simulink model "dynamicsquat"  (R2023a)
settings: Solver=VariableStepAuto  StartTime=0.0  StopTime=stoptimetotal  RelTol=1e-3
values from neighbouring files (symbols this model uses):
  battery = load('params/battery_Tattu.mat').battery    [runDetailedT18Model.m]
  IC = load('params/initialcond/IC_HoverAt30mOcto.mat').IC    [runDetailedT18Model.m]
  maxleashvelocity = 5    [runDetailedT18Model.m]
  Motor = load('params/KDE4213XF-360_performancedata.mat').Motor    [runDetailedT18Model.m]
  octomodel = load('params/TarotT18.mat').octomodel    [runDetailedT18Model.m]
  turbenabled = 0    [runDetailedT18Model.m]
  xref = xyzref(waypts,1)    [runDetailedT18Model.m]
  yref = xyzref(waypts,2)    [runDetailedT18Model.m]
  zref = xyzref(waypts,3)    [runDetailedT18Model.m]
undefined symbols (not defined in the file or in its folder): deg, DiscIntNeverNeededParam, F, Light, MIL, rad, s
libraries: aerolibconvert2 x2, shared6dof x1, aerolibwind2 x1
(part 1 of 2)
settings Model: PacingRate=9  Creator=Researcher  LastModifiedBy=abenezertaye
settings SolverCC: ZeroCrossAlgorithm=Adaptive  AlgebraicLoopSolver=TrustRegion
settings DataIOCC: ReturnWorkspaceOutputs=off
settings OptimizationCC: ReuseModelBlockBuffer=off
settings DebuggingCC: IgnoredZcDiagnostic=none  UnconnectedInputMsg=warning  UnconnectedOutputMsg=warning  UnconnectedLineMsg=warning  ArithmeticOperatorsInVariantConditions=warning
settings ModelReferenceCC: EnableRefExpFcnMdlSchedulingChecks=on
settings SFSimCC: SimUseLocalCustomCode=off  CustomCodeUndefinedFunction=UseInterfaceOnly
settings RTWCC: RTWUseLocalCustomCode=off  DLArmComputeVersion=19.05

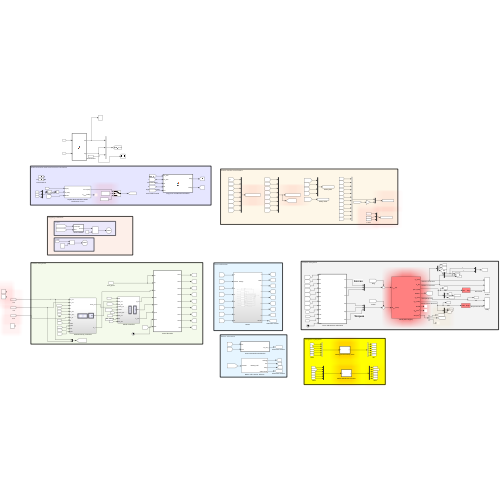
[thumbnail: Simulink's stored preview of the top-level diagram]
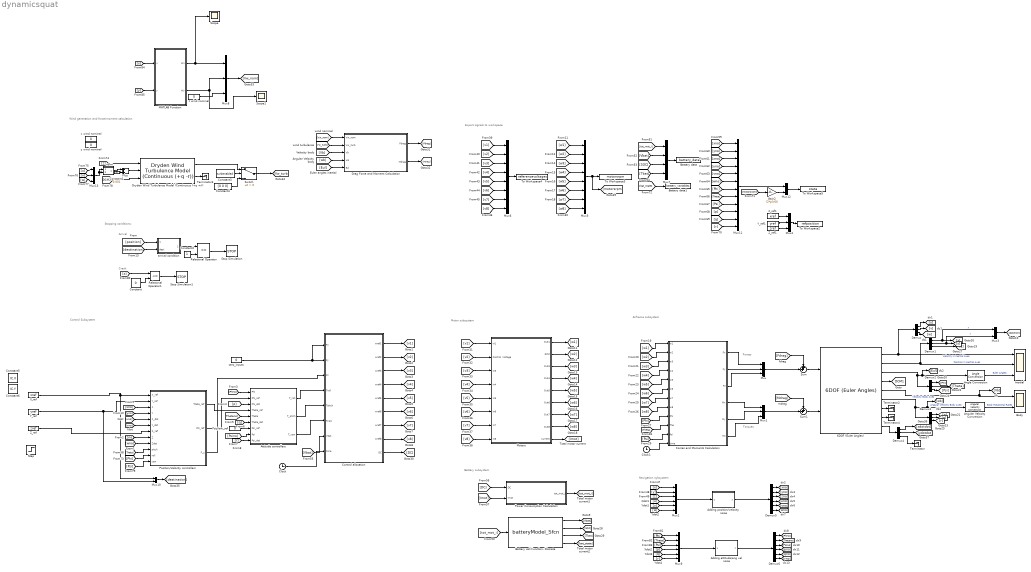
== system dynamicsquat ==
  note: Navigation sybsystem
  note: Airframe subsystem
  note: Motor subsystem
  note: Control Subsystem
  note: Battery subsystem
  note: Export signals to workspace
  note: Wind generation and force/moment calculation
  note: Forces
  note: Torques
  note: Stopping conditions:
  note: Crash
  note: Arrival
  6DOF (Euler Angles) : shared6dof/6DOF (Euler Angles)  units=Metric (MKS)  mtype=Fixed  rep=Quaternion  xme_0=[IC.X IC.Y IC.Z]  Vm_0=[0 0 0]  eul_0=[0 0 0]  pm_0=[0 0 0]  mass_0=octomodel.mass  mass_e=0.5  mass_f=2.0  inertia=octomodel.Jb  inertia_e=eye(3)  inertia_f=2*eye(3)  k_quat=1.0  vre_flag=on  abi_flag=on  aMode=0  xme_statename=''  Vm_statename=''  eul_statename=''  quat_statename=''  pm_statename=''  mass_statename=''
  Adding attitude/ang vel noise : MATLAB Function  TreatAsAtomicUnit=on  SystemSampleTime=octomodel.sampletime
  Adding position/velocity noise : MATLAB Function  TreatAsAtomicUnit=on  SystemSampleTime=octomodel.sampletime
  Angle Conversion : aerolibconvert2/Angle Conversion  IU=rad  OU=deg
  Angular Velocity Conversion : aerolibconvert2/Angular Velocity Conversion  IU=rad/s  OU=deg/s
  Attitude controllers : Subsystem
  Battery cell Function- Discrete : M-S-Function  FunctionName=batteryModel_Sfcn  Parameters=battery
      mask Display:
      | port_label('input', 1, 'current');
      | port_label('output', 1, 'voltage');
      | port_label('output', 2, 'soc');
      | port_label('output', 3, 'temp');
      | port_label('output', 4, 'state vector');
      | 
      | disp("Battery Cell");
  Battery data : ToWorkspace  VariableName=battery_data  SaveFormat=Timeseries  SampleTime=battery.sampleTime
  Battery data1 : ToWorkspace  VariableName=battery_variables  SaveFormat=Timeseries  SampleTime=battery.sampleTime
  Body : Scope  NumInputPorts=2
  Clock : Clock
  Clock1 : Clock
  Constant : Constant  Value=0
  Constant1 : Constant  Value=0.001
  Constant2 : Constant
  Constant3 : Constant  Value=turbenabled
  Constant4 : Constant  Value=[0 0 0]
  Constant5 : Constant  Value=IC.X
  Constant6 : Constant  Value=IC.Y
  Control allocation : MATLAB Function  TreatAsAtomicUnit=on
  Demux{,1..4} (5 alike) : Demux  Outputs=3
  Demux5 : Demux  Outputs=6
  Demux6 : Demux  Outputs=6
  Drag Force and Moment Calculation : MATLAB Function  TreatAsAtomicUnit=on
  Dryden Wind Turbulence Model (Continuous (+q +r)) : aerolibwind2/Dryden Wind Turbulence Model  (Continuous (+q -r))  units=Metric (MKS)  spec=MIL-F-8785C  model=Continuous Dryden (+q +r)  W20=15  Wdeg=0  TurbProb=10^-2 - Light  L_high=533.4  Wingspan=10  ts=0.1  Seed=[23341 23342 23343 23344]  T_on=on
      settings: LibrarySourceBlock=|
      | aerolibwind2/Dryden Wind Turbulence Model
      | (Continuous (+q +r))
  Forces and Moments Calculation : MATLAB Function  TreatAsAtomicUnit=on
  Gain2 : Gain  Gain=(2*pi)/60
  Inertial : Scope  NumInputPorts=3
  MATLAB Function : MATLAB Function  TreatAsAtomicUnit=on
  Motors : Subsystem
  Mux{,1,4,8,13} (5 alike) : Mux  Inputs=3
  Mux10 : Mux  Inputs=2
  Mux11 : Mux  Inputs=12
  Mux12 : Mux  Inputs=2
  Mux2 : Mux  Inputs=6
  Mux3 : Mux  Inputs=2
  Mux5 : Mux  Inputs=8
  Mux6 : Mux  Inputs=8
  Mux7 : Mux
  Mux9 : Mux  Inputs=6
  Plus : Sum
  Position/Velocity controllers : Subsystem
  Power Consumption Calculation : MATLAB Function  TreatAsAtomicUnit=on
  Psi_Yaw_ref : Constant  Value=0
  Relational Operator : RelationalOperator  Operator===  OutDataTypeStr=boolean  RndMeth=Simplest  InputSameDT=off
  Relational Operator1 : RelationalOperator  Operator=<=  OutDataTypeStr=boolean  RndMeth=Simplest  InputSameDT=off
  Scope : Scope
  Scope1 : Scope
  Step : Step  Before=IC.Z  After=IC.Z+5  SampleTime=0
  Stop Simulation : Stop
  Stop Simulation1 : Stop
  Sum : Sum  Inputs=++|
  Sum1 : Sum  Inputs=++|
  Switch : Switch  Criteria=u2 > Threshold  SaturateOnIntegerOverflow=off  InputSameDT=off
  Terminator{,2..4} (4 alike) : Terminator
  To Workspace2 : ToWorkspace  VariableName=refposition  SaveFormat=Timeseries  SampleTime=octomodel.sampletime
  To Workspace3 : ToWorkspace  VariableName=motorsrpm  SaveFormat=Timeseries  SampleTime=octomodel.sampletime
  To Workspace4 : ToWorkspace  VariableName=referencevoltages  SaveFormat=Timeseries  SampleTime=octomodel.sampletime
  To Workspace5 : ToWorkspace  VariableName=state  SaveFormat=Timeseries  SampleTime=octomodel.sampletime
  X_ref : Constant  Value=xref
  X_ref1 : Constant  Value=xref
  Y_ref : Constant  Value=yref
  Y_ref1 : Constant  Value=yref
  Z_ref : Constant  Value=zref
  Z_ref1 : Constant  Value=zref
  arrival condition : MATLAB Function  TreatAsAtomicUnit=on
  norm : Subsystem
  x wind nominal : Constant  Value=0
  y wind nominal : Constant  Value=0
  z wind nominal : Constant  Value=0
  zero_inputs : Constant  Value=0
  tag scope: DCM1=global
  wires:
  zero_inputs/1 -> Control allocation/1(Fx), Control allocation/2(Fy)
  [yno] -> Position/Velocity controllers/4(Y)
  [xno] -> Position/Velocity controllers/3(X)
  [Phino] -> Attitude controllers/1(Phi)
  [p] -> Attitude controllers/3(Phi_dot)
  [Thetano] -> Attitude controllers/5(Theta)
  [q] -> Attitude controllers/6(Theta_dot)
  Psi_Yaw_ref/1 -> Attitude controllers/7(Psi_ref)
  [Psino] -> Attitude controllers/8(Psi)
  [r] -> Attitude controllers/9(Psi_dot)
  Motors/9(current) -> [Imot]
  Motors/8(Out8) -> [w8]
  Motors/1(Out1) -> [w1]
  Motors/2(RPM) -> [w2]
  Motors/7(Out7) -> [w7]
  Motors/6(Out6) -> [w6]
  Motors/5(Out5) -> [w5]
  Motors/3(Out3) -> [w3]
  Motors/4(Out4) -> [w4]
  Mux1/1 -> Sum1/2
  Mux/1 -> Sum/2
  [Phi] -> Forces and Moments Calculation/9(Phi)
  [Theta] -> Forces and Moments Calculation/10(The)
  [Psi] -> Forces and Moments Calculation/11(Psi)
  6DOF (Euler Angles)/8 -> Terminator4/1
  6DOF (Euler Angles)/7 -> Terminator2/1
  6DOF (Euler Angles)/6 -> Demux3/1, [wb], Angular Velocity Conversion/1  "Angular Velocity Body Axes"
  6DOF (Euler Angles)/4 -> [DCM1]
  6DOF (Euler Angles)/2 -> Inertial/2, Demux1/1  "Position in Inertial Axes"
  Angle Conversion/1 -> Inertial/3  "Euler Angles"
  Angular Velocity Conversion/1 -> Body/2  "Body Rotational Rates"
  6DOF (Euler Angles)/1 -> Demux/1, Inertial/1  "Velocity in Inertial Axes"
  6DOF (Euler Angles)/3 -> Demux2/1, [Eul], Angle Conversion/1
  6DOF (Euler Angles)/5 -> Body/1, [Vb]  "Velocity Body Axes"
  Demux1/3 -> [z]
  Demux/3 -> [w]
  Demux/2 -> [v]
  Demux/1 -> [u]
  Demux2/3 -> [Psi]
  Demux2/2 -> [Theta]
  Demux2/1 -> [Phi]
  Demux3/1 -> [p]
  Demux3/2 -> [q]
  Demux3/3 -> [r]
  Demux1/2 -> Mux3/2, [y]  "y"
  Mux3/1 -> [position]
  Demux1/1 -> Mux3/1, [x]  "x"
  Mux5/1 -> [motorsrpm], To Workspace3/1
  [w8] -> Mux5/8
  [w5] -> Mux5/5
  [w4] -> Mux5/4
  [w1] -> Mux5/1
  [w7] -> Mux5/7
  [w3] -> Mux5/3
  [w2] -> Mux5/2
  [w6] -> Mux5/6
  Control allocation/5(wref5) -> [v5]
  Control allocation/6(wref6) -> [v6]
  Control allocation/4(wref4) -> [v4]
  Control allocation/3(wref3) -> [v3]
  Control allocation/2(wref2) -> [v2]
  Control allocation/8(wref8) -> [v8]
  Control allocation/7(wref7) -> [v7]
  Control allocation/1(wref1) -> [v1]
  [v8] -> Motors/8(In8)
  [v5] -> Motors/5(In5)
  [v4] -> Motors/4(In4)
  [v1] -> Motors/1(In1)
  [v7] -> Motors/7(In7)
  [v3] -> Motors/3(In3)
  [v2] -> Motors/2(Control  Voltage)
  [v6] -> Motors/6(In6)
  [v2] -> Mux6/2
  [v7] -> Mux6/7
  [v8] -> Mux6/8
  [v4] -> Mux6/4
  Mux6/1 -> To Workspace4/1
  [v5] -> Mux6/5
  [v6] -> Mux6/6
  [v3] -> Mux6/3
  [v1] -> Mux6/1
  Battery cell Function- Discrete/2 -> [SOC]
  Battery cell Function- Discrete/1 -> [Vbat]
  Battery cell Function- Discrete/3 -> [Tbat]
  Mux7/1 -> Battery data/1
  [tot_mot_i] -> Battery cell Function- Discrete/1
  [tot_mot_i] -> Mux7/1
  [Vbat] -> Mux7/2
  [SOC] -> Mux7/3
  [Tbat] -> Mux7/4
  [Vbat] -> Control allocation/7(Vbat)
  Control allocation/9(DC) -> [DC]
  [DC] -> Power Consumption Calculation/1(DC)
  Power Consumption Calculation/1(tot_mot_i) -> [tot_mot_i]
  [Imot] -> Power Consumption Calculation/2(Imot)
  [Vw_nom] -> Drag Force and Moment Calculation/1(Vw_nom)
  [Vw_turb] -> Drag Force and Moment Calculation/2(Vw_turb)
  [Vb] -> Drag Force and Moment Calculation/3(Vb)
  [wb] -> Drag Force and Moment Calculation/4(wb)
  Sum/1 -> 6DOF (Euler Angles)/1
  Sum1/1 -> 6DOF (Euler Angles)/2
  [Mdrag] -> Sum1/1
  [Fdrag] -> Sum/1
  Drag Force and Moment Calculation/2(Mdrag) -> [Mdrag]
  Drag Force and Moment Calculation/1(Fdrag) -> [Fdrag]
  [Eul] -> Drag Force and Moment Calculation/5(Eul)
  z wind nominal/1 -> Mux8/3
  Mux10/1 -> [destination]
  X_ref/1 -> Mux10/1, Position/Velocity controllers/1(X_ref)
  Y_ref/1 -> Mux10/2, Position/Velocity controllers/2(Y_ref)
  [uno] -> Position/Velocity controllers/5(X_dot)
  [vno] -> Position/Velocity controllers/6(Y_dot)
  Demux4/2 -> [ydotdot]
  6DOF (Euler Angles)/9 -> Demux4/1
  Demux4/1 -> [xdotdot]
  Demux4/3 -> Terminator/1
  Attitude controllers/3(T_yaw) -> Control allocation/6(Tyaw)
  Attitude controllers/2(T_pitch) -> Control allocation/5(Tpitch)
  Position/Velocity controllers/2(Phi_ref) -> Attitude controllers/2(Phi_ref)
  Mux11/1 -> Mux12/1
  [xno] -> Mux11/1
  [yno] -> Mux11/2
  [zno] -> Mux11/3
  [uno] -> Mux11/4
  [vno] -> Mux11/5
  [wno] -> Mux11/6
  [Phi] -> Mux11/7
  [Theta] -> Mux11/8
  [Psi] -> Mux11/9
  [p] -> Mux11/10
  [q] -> Mux11/11
  [r] -> Mux11/12
  Mux12/1 -> To Workspace5/1
  [motorsrpm] -> Gain2/1
  Gain2/1 -> Mux12/2
  [bat_state] -> Battery data1/1
  Battery cell Function- Discrete/4 -> [bat_state]
  Position/Velocity controllers/3(F_z) -> Control allocation/3(Fz)
  [x] -> Mux2/1
  [z] -> Mux2/3
  [v] -> Mux2/5
  [y] -> Mux2/2
  Mux2/1 -> Adding position/velocity noise/1(u)
  [w] -> Mux2/6
  [u] -> Mux2/4
  Demux5/1 -> [xno]
  Demux5/2 -> [yno]
  Demux5/3 -> [zno]
  Demux5/4 -> [uno]
  Demux5/5 -> [vno]
  Demux5/6 -> [wno]
  [z] -> Dryden Wind Turbulence Model (Continuous (+q +r))/1
  [w] -> Mux13/3
  [v] -> Mux13/2
  [u] -> Mux13/1
  Mux13/1 -> norm/1(In1), norm/2(In2)
  norm/1(Out1) -> Plus/1
  [DCM1] -> Dryden Wind Turbulence Model (Continuous (+q +r))/3
  Dryden Wind Turbulence Model (Continuous (+q +r))/2 -> Terminator3/1
  Plus/1 -> Dryden Wind Turbulence Model (Continuous (+q +r))/2
  Constant1/1 -> Plus/2
  Constant3/1 -> Switch/2
  Dryden Wind Turbulence Model (Continuous (+q +r))/1 -> Switch/1
  Constant4/1 -> Switch/3
  Switch/1 -> [Vw_turb]
  Attitude controllers/1(T_roll) -> Control allocation/4(Troll)
  Forces and Moments Calculation/1(Fx) -> Mux/1
  Forces and Moments Calculation/2(Fy) -> Mux/2
  Forces and Moments Calculation/3(Fz) -> Mux/3
  Forces and Moments Calculation/4(Mx) -> Mux1/1
  Forces and Moments Calculation/5(My) -> Mux1/2
  Forces and Moments Calculation/6(Mz) -> Mux1/3
  Clock/1 -> Control allocation/8(time)
  [w1] -> Forces and Moments Calculation/1(w1)
  [w2] -> Forces and Moments Calculation/2(w2)
  [w3] -> Forces and Moments Calculation/3(w3)
  [w4] -> Forces and Moments Calculation/4(w4)
  [w5] -> Forces and Moments Calculation/5(w5)
  [w6] -> Forces and Moments Calculation/6(w6)
  [w7] -> Forces and Moments Calculation/7(w7)
  [w8] -> Forces and Moments Calculation/8(w8)
  Clock1/1 -> Forces and Moments Calculation/12(time)
  Position/Velocity controllers/1(Theta_ref) -> Attitude controllers/4(Theta_ref)
  Z_ref/1 -> Position/Velocity controllers/7(Z_ref)
  [zno] -> Position/Velocity controllers/8(Z)
  [wno] -> Position/Velocity controllers/9(Zdot)
  [Theta] -> Position/Velocity controllers/10(pitch)
  [Phi] -> Position/Velocity controllers/11(roll)
  [Psi] -> Position/Velocity controllers/12(yaw)
  Adding position/velocity noise/1(y) -> Demux5/1
  Adding attitude/ang vel noise/1(y) -> Demux6/1
  Demux6/6 -> [rno]
  Demux6/5 -> [qno]
  Demux6/4 -> [pno]
  Demux6/3 -> [Psino]
  Demux6/2 -> [Thetano]
  Demux6/1 -> [Phino]
  [p] -> Mux9/4
  [r] -> Mux9/6
  Mux9/1 -> Adding attitude/ang vel noise/1(u)
  [Theta] -> Mux9/2
  [q] -> Mux9/5
  [Psi] -> Mux9/3
  [Phi] -> Mux9/1
  [z] -> Relational Operator1/1
  Constant2/1 -> Relational Operator/2
  Relational Operator/1 -> Stop Simulation/1
  Constant/1 -> Relational Operator1/2
  [position] -> arrival condition/1(currentpos)
  arrival condition/1(arrived) -> Relational Operator/1
  [destination] -> arrival condition/2(dest)
  Relational Operator1/1 -> Stop Simulation1/1
  X_ref1/1 -> Mux4/1
  Y_ref1/1 -> Mux4/2
  Z_ref1/1 -> Mux4/3
  Mux4/1 -> To Workspace2/1
  Mux8/1 -> [Vw_nom]
  MATLAB Function/1(Wx) -> Mux8/1, Scope/1
  MATLAB Function/2(Wy) -> Mux8/2, Scope1/1
  [x] -> MATLAB Function/1(x)
  [y] -> MATLAB Function/2(y)

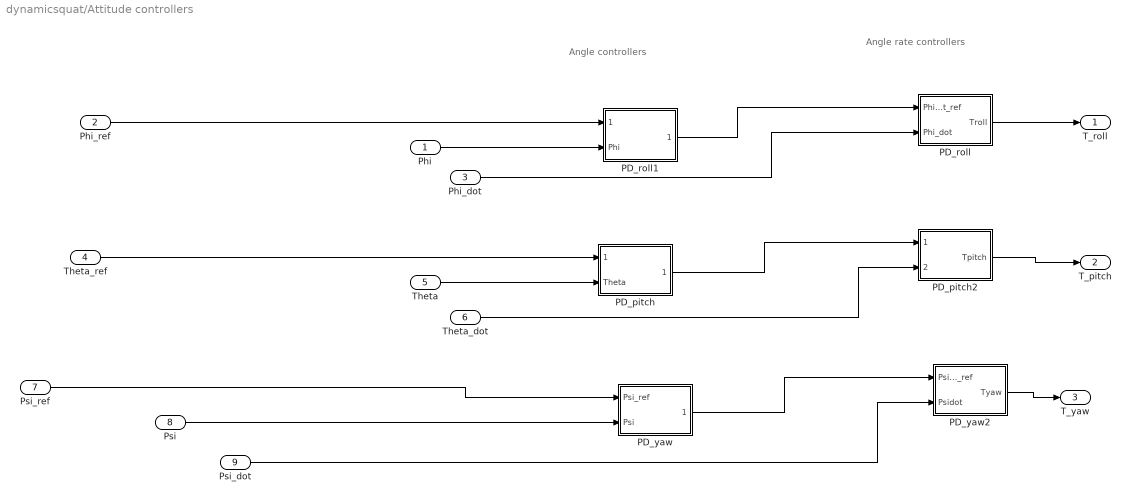
== system dynamicsquat/Attitude controllers ==
  note: Angle rate controllers
  note: Angle controllers
  Phi : Inport
  Phi_ref : Inport  Port=2
  Phi_dot : Inport  Port=3
  Theta_ref : Inport  Port=4
  Theta : Inport  Port=5
  Theta_dot : Inport  Port=6
  Psi_ref : Inport  Port=7
  Psi : Inport  Port=8
  Psi_dot : Inport  Port=9
  PD_pitch : Subsystem
  PD_pitch2 : Subsystem
  PD_roll : Subsystem
  PD_roll1 : Subsystem
  PD_yaw : Subsystem
  PD_yaw2 : Subsystem
  T_roll : Outport  VectorParamsAs1DForOutWhenUnconnected=off
  T_pitch : Outport  Port=2  VectorParamsAs1DForOutWhenUnconnected=off
  T_yaw : Outport  Port=3  VectorParamsAs1DForOutWhenUnconnected=off
  wires:
  PD_roll/1(Troll) -> T_roll/1
  Phi/1 -> PD_roll1/2(Phi)
  Phi_dot/1 -> PD_roll/2(Phi_dot)
  Theta_dot/1 -> PD_pitch2/2(Thetadot)
  Theta/1 -> PD_pitch/2(Theta)
  PD_pitch2/1(Tpitch) -> T_pitch/1
  Psi_dot/1 -> PD_yaw2/2(Psidot)
  PD_yaw2/1(Tyaw) -> T_yaw/1
  Psi/1 -> PD_yaw/2(Psi)
  Phi_ref/1 -> PD_roll1/1(Phi_ref)
  PD_roll1/1(Phidot_ref) -> PD_roll/1(Phidot_ref)
  PD_yaw/1(Psidot_ref) -> PD_yaw2/1(Psidot_ref)
  PD_pitch/1(Thetadot_ref) -> PD_pitch2/1(Thetadot_ref)
  Theta_ref/1 -> PD_pitch/1(Theta_ref)
  Psi_ref/1 -> PD_yaw/1(Psi_ref)

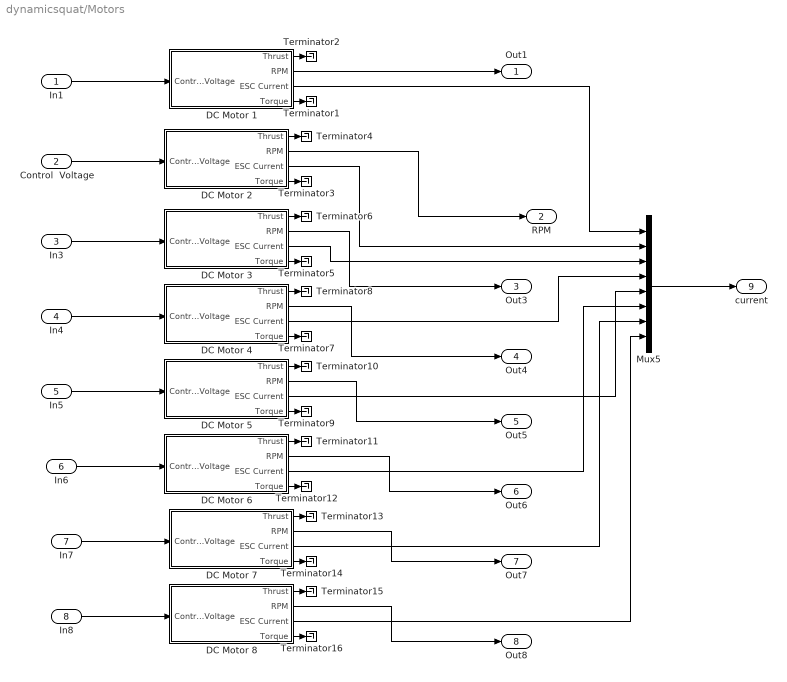
== system dynamicsquat/Motors ==
  In1 : Inport
  Control  Voltage : Inport  Port=2
  In3 : Inport  Port=3
  In4 : Inport  Port=4
  In5 : Inport  Port=5
  In6 : Inport  Port=6
  In7 : Inport  Port=7
  In8 : Inport  Port=8
  DC Motor 1 : Subsystem
  DC Motor 2 : Subsystem
  DC Motor 3 : Subsystem
  DC Motor 4 : Subsystem
  DC Motor 5 : Subsystem
  DC Motor 6 : Subsystem
  DC Motor 7 : Subsystem
  DC Motor 8 : Subsystem
  Mux5 : Mux  Inputs=8
  Terminator{1..16} (16 alike) : Terminator
  Out1 : Outport  VectorParamsAs1DForOutWhenUnconnected=off
  RPM : Outport  Port=2  VectorParamsAs1DForOutWhenUnconnected=off
  Out3 : Outport  Port=3  VectorParamsAs1DForOutWhenUnconnected=off
  Out4 : Outport  Port=4  VectorParamsAs1DForOutWhenUnconnected=off
  Out5 : Outport  Port=5  VectorParamsAs1DForOutWhenUnconnected=off
  Out6 : Outport  Port=6  VectorParamsAs1DForOutWhenUnconnected=off
  Out7 : Outport  Port=7  VectorParamsAs1DForOutWhenUnconnected=off
  Out8 : Outport  Port=8  VectorParamsAs1DForOutWhenUnconnected=off
  current : Outport  Port=9  VectorParamsAs1DForOutWhenUnconnected=off
  wires:
  DC Motor 6/3(ESC Current) -> Mux5/6
  DC Motor 7/3(ESC Current) -> Mux5/7
  DC Motor 5/3(ESC Current) -> Mux5/5
  DC Motor 8/3(ESC Current) -> Mux5/8
  DC Motor 1/3(ESC Current) -> Mux5/1
  DC Motor 2/3(ESC Current) -> Mux5/2
  DC Motor 4/3(ESC Current) -> Mux5/4
  DC Motor 3/3(ESC Current) -> Mux5/3
  DC Motor 5/2(RPM) -> Out5/1
  DC Motor 7/2(RPM) -> Out7/1
  DC Motor 3/2(RPM) -> Out3/1
  DC Motor 4/2(RPM) -> Out4/1
  DC Motor 6/2(RPM) -> Out6/1
  DC Motor 8/2(RPM) -> Out8/1
  DC Motor 1/2(RPM) -> Out1/1
  In7/1 -> DC Motor 7/1(Control Voltage)
  In8/1 -> DC Motor 8/1(Control Voltage)
  In6/1 -> DC Motor 6/1(Control Voltage)
  In5/1 -> DC Motor 5/1(Control Voltage)
  In4/1 -> DC Motor 4/1(Control Voltage)
  In3/1 -> DC Motor 3/1(Control Voltage)
  Control  Voltage/1 -> DC Motor 2/1(Control Voltage)
  Mux5/1 -> current/1
  DC Motor 1/1(Thrust) -> Terminator2/1
  DC Motor 1/4(Torque) -> Terminator1/1
  DC Motor 2/4(Torque) -> Terminator3/1
  DC Motor 2/1(Thrust) -> Terminator4/1
  DC Motor 3/1(Thrust) -> Terminator6/1
  DC Motor 3/4(Torque) -> Terminator5/1
  DC Motor 4/4(Torque) -> Terminator7/1
  DC Motor 4/1(Thrust) -> Terminator8/1
  DC Motor 5/1(Thrust) -> Terminator10/1
  DC Motor 5/4(Torque) -> Terminator9/1
  DC Motor 6/4(Torque) -> Terminator12/1
  DC Motor 6/1(Thrust) -> Terminator11/1
  DC Motor 7/1(Thrust) -> Terminator13/1
  DC Motor 7/4(Torque) -> Terminator14/1
  DC Motor 8/4(Torque) -> Terminator16/1
  DC Motor 8/1(Thrust) -> Terminator15/1
  In1/1 -> DC Motor 1/1(Control Voltage)
  DC Motor 2/2(RPM) -> RPM/1

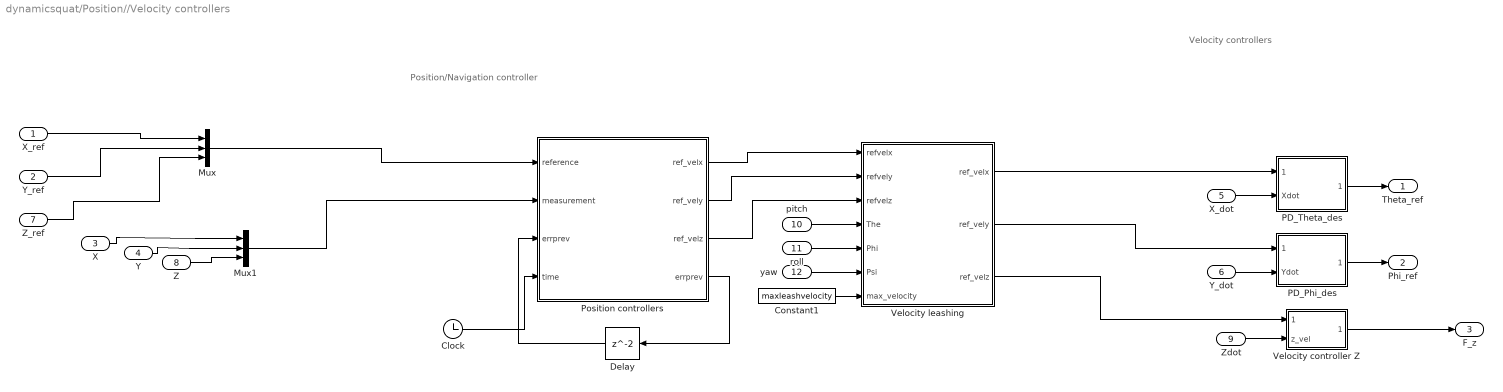
== system dynamicsquat/Position//Velocity controllers ==
  note: Position/Navigation controller
  note: Velocity controllers
  X_ref : Inport
  Y_ref : Inport  Port=2
  X : Inport  Port=3
  Y : Inport  Port=4
  X_dot : Inport  Port=5
  Y_dot : Inport  Port=6
  Z_ref : Inport  Port=7
  Z : Inport  Port=8
  Zdot : Inport  Port=9
  pitch : Inport  Port=10
  roll : Inport  Port=11
  yaw : Inport  Port=12
  Clock : Clock
  Constant1 : Constant  Value=maxleashvelocity
  Delay : Delay  SampleTime=0.01
  Mux : Mux  Inputs=3
  Mux1 : Mux  Inputs=3
  PD_Phi_des : Subsystem
  PD_Theta_des : Subsystem
  Position controllers : MATLAB Function  TreatAsAtomicUnit=on
  Velocity controller Z : Subsystem
  Velocity leashing : MATLAB Function  TreatAsAtomicUnit=on
  Theta_ref : Outport  VectorParamsAs1DForOutWhenUnconnected=off
  Phi_ref : Outport  Port=2  VectorParamsAs1DForOutWhenUnconnected=off
  F_z : Outport  Port=3  VectorParamsAs1DForOutWhenUnconnected=off
  wires:
  X/1 -> Mux1/1
  PD_Phi_des/1(Phi_ref) -> Phi_ref/1
  PD_Theta_des/1(Theta_ref) -> Theta_ref/1
  Y_dot/1 -> PD_Phi_des/2(Ydot)
  Y/1 -> Mux1/2
  Mux/1 -> Position controllers/1(reference)
  Mux1/1 -> Position controllers/2(measurement)
  Position controllers/4(errprev) -> Delay/1
  Delay/1 -> Position controllers/3("errprev ")
  Constant1/1 -> Velocity leashing/7(max_velocity)
  X_dot/1 -> PD_Theta_des/2(Xdot)
  Velocity controller Z/1(Thrust) -> F_z/1
  Zdot/1 -> Velocity controller Z/2(z_vel)
  Z/1 -> Mux1/3
  Position controllers/1(ref_velx) -> Velocity leashing/1(refvelx)
  Position controllers/3(ref_velz) -> Velocity leashing/3(refvelz)
  pitch/1 -> Velocity leashing/4(The)
  roll/1 -> Velocity leashing/5(Phi)
  yaw/1 -> Velocity leashing/6(Psi)
  Velocity leashing/1(ref_velx) -> PD_Theta_des/1(Xdot_ref)
  Velocity leashing/2(ref_vely) -> PD_Phi_des/1(Ydot_ref)
  Velocity leashing/3(ref_velz) -> Velocity controller Z/1(z_velref)
  Position controllers/2(ref_vely) -> Velocity leashing/2(refvely)
  X_ref/1 -> Mux/1
  Y_ref/1 -> Mux/2
  Clock/1 -> Position controllers/4(time)
  Z_ref/1 -> Mux/3

== system dynamicsquat/norm ==
  In1 : Inport
  In2 : Inport  Port=2
  Dot Product : DotProduct  OutDataTypeStr=Inherit: Inherit via internal rule
  Sqrt : Sqrt
  Out1 : Outport
  wires:
  Dot Product/1 -> Sqrt/1
  In1/1 -> Dot Product/1
  In2/1 -> Dot Product/2
  Sqrt/1 -> Out1/1

== system dynamicsquat/Attitude controllers/PD_pitch ==
  Theta_ref : Inport
  Theta : Inport  Port=2
  Add : Sum  Inputs=+-
  Gain : Gain  Gain=5
  Scope : Scope  NumInputPorts=2
  Thetadot_ref : Outport  VectorParamsAs1DForOutWhenUnconnected=off
  wires:
  Theta_ref/1 -> Scope/1, Add/1
  Add/1 -> Gain/1
  Theta/1 -> Scope/2, Add/2
  Gain/1 -> Thetadot_ref/1

== system dynamicsquat/Attitude controllers/PD_pitch2 ==
  Thetadot_ref : Inport
  Thetadot : Inport  Port=2
  Add : Sum  Inputs=+-
  Gain : Gain  Gain=8
  Tpitch : Outport  VectorParamsAs1DForOutWhenUnconnected=off
  wires:
  Thetadot/1 -> Add/2
  Add/1 -> Gain/1
  Thetadot_ref/1 -> Add/1
  Gain/1 -> Tpitch/1

== system dynamicsquat/Attitude controllers/PD_roll ==
  Phidot_ref : Inport
  Phi_dot : Inport  Port=2
  Add : Sum  Inputs=+-
  Gain : Gain  Gain=8
  Troll : Outport  VectorParamsAs1DForOutWhenUnconnected=off
  wires:
  Add/1 -> Gain/1
  Gain/1 -> Troll/1
  Phi_dot/1 -> Add/2
  Phidot_ref/1 -> Add/1

== system dynamicsquat/Attitude controllers/PD_roll1 ==
  Phi_ref : Inport
  Phi : Inport  Port=2
  Add : Sum  Inputs=+-
  Gain : Gain  Gain=5
  Phidot_ref : Outport  VectorParamsAs1DForOutWhenUnconnected=off
  wires:
  Add/1 -> Gain/1
  Phi/1 -> Add/2
  Phi_ref/1 -> Add/1
  Gain/1 -> Phidot_ref/1

== system dynamicsquat/Attitude controllers/PD_yaw ==
  Psi_ref : Inport
  Psi : Inport  Port=2
  Add : Sum  Inputs=+-
  Gain : Gain  Gain=5
  Psidot_ref : Outport  VectorParamsAs1DForOutWhenUnconnected=off
  wires:
  Psi_ref/1 -> Add/1
  Add/1 -> Gain/1
  Psi/1 -> Add/2
  Gain/1 -> Psidot_ref/1

== system dynamicsquat/Attitude controllers/PD_yaw2 ==
  Psidot_ref : Inport
  Psidot : Inport  Port=2
  Add : Sum  Inputs=+-
  Gain : Gain  Gain=8
  Tyaw : Outport  VectorParamsAs1DForOutWhenUnconnected=off
  wires:
  Gain/1 -> Tyaw/1
  Psidot/1 -> Add/2
  Add/1 -> Gain/1
  Psidot_ref/1 -> Add/1

== system dynamicsquat/Motors/DC Motor 1 ==
  Control Voltage : Inport
  Convert rad/s to rmp : Gain  Gain=60/(2*pi)
  Electrical part : Subsystem
  Mechanical part : Subsystem
  StaticTfric : Constant  Value=0
  Thrust : Outport  VectorParamsAs1DForOutWhenUnconnected=off
  RPM : Outport  Port=2  VectorParamsAs1DForOutWhenUnconnected=off
  ESC Current : Outport  Port=3  VectorParamsAs1DForOutWhenUnconnected=off
  Torque : Outport  Port=4  VectorParamsAs1DForOutWhenUnconnected=off
  wires:
  StaticTfric/1 -> Mechanical part/1(Static Friction Torque)
  Convert rad/s to rmp/1 -> RPM/1
  Electrical part/1(Electrical Torque) -> Mechanical part/2(Electrical Torque)
  Mechanical part/1(w angular speed) -> Electrical part/2(w angular speed), Convert rad/s to rmp/1
  Mechanical part/2(Thrust) -> Thrust/1
  Electrical part/2(current) -> ESC Current/1
  Control Voltage/1 -> Electrical part/1(ESC voltage)
  Mechanical part/3(Torque) -> Torque/1

== system dynamicsquat/Motors/DC Motor 2 ==
  Control Voltage : Inport
  Convert rad/s to rmp : Gain  Gain=60/(2*pi)
  Electrical part : Subsystem
  Mechanical part : Subsystem
  StaticTfric : Constant  Value=0
  Thrust : Outport  VectorParamsAs1DForOutWhenUnconnected=off
  RPM : Outport  Port=2  VectorParamsAs1DForOutWhenUnconnected=off
  ESC Current : Outport  Port=3  VectorParamsAs1DForOutWhenUnconnected=off
  Torque : Outport  Port=4  VectorParamsAs1DForOutWhenUnconnected=off
  wires:
  Mechanical part/3(Torque) -> Torque/1
  Control Voltage/1 -> Electrical part/1(ESC voltage)
  Electrical part/2(current) -> ESC Current/1
  Mechanical part/2(Thrust) -> Thrust/1
  Mechanical part/1(w angular speed) -> Convert rad/s to rmp/1, Electrical part/2(w angular speed)
  Electrical part/1(Electrical Torque) -> Mechanical part/2(Electrical Torque)
  Convert rad/s to rmp/1 -> RPM/1
  StaticTfric/1 -> Mechanical part/1(Static Friction Torque)

== system dynamicsquat/Motors/DC Motor 3 ==
  Control Voltage : Inport
  Convert rad/s to rmp : Gain  Gain=60/(2*pi)
  Electrical part : Subsystem
  Mechanical part : Subsystem
  StaticTfric : Constant  Value=0
  Thrust : Outport  VectorParamsAs1DForOutWhenUnconnected=off
  RPM : Outport  Port=2  VectorParamsAs1DForOutWhenUnconnected=off
  ESC Current : Outport  Port=3  VectorParamsAs1DForOutWhenUnconnected=off
  Torque : Outport  Port=4  VectorParamsAs1DForOutWhenUnconnected=off
  wires:
  StaticTfric/1 -> Mechanical part/1(Static Friction Torque)
  Convert rad/s to rmp/1 -> RPM/1
  Electrical part/1(Electrical Torque) -> Mechanical part/2(Electrical Torque)
  Mechanical part/1(w angular speed) -> Electrical part/2(w angular speed), Convert rad/s to rmp/1
  Mechanical part/2(Thrust) -> Thrust/1
  Electrical part/2(current) -> ESC Current/1
  Control Voltage/1 -> Electrical part/1(ESC voltage)
  Mechanical part/3(Torque) -> Torque/1

== system dynamicsquat/Motors/DC Motor 4 ==
  Control Voltage : Inport
  Convert rad/s to rmp : Gain  Gain=60/(2*pi)
  Electrical part : Subsystem
  Mechanical part : Subsystem
  StaticTfric : Constant  Value=0
  Thrust : Outport  VectorParamsAs1DForOutWhenUnconnected=off
  RPM : Outport  Port=2  VectorParamsAs1DForOutWhenUnconnected=off
  ESC Current : Outport  Port=3  VectorParamsAs1DForOutWhenUnconnected=off
  Torque : Outport  Port=4  VectorParamsAs1DForOutWhenUnconnected=off
  wires:
  Mechanical part/3(Torque) -> Torque/1
  Control Voltage/1 -> Electrical part/1(ESC voltage)
  Electrical part/2(current) -> ESC Current/1
  Mechanical part/2(Thrust) -> Thrust/1
  Mechanical part/1(w angular speed) -> Convert rad/s to rmp/1, Electrical part/2(w angular speed)
  Electrical part/1(Electrical Torque) -> Mechanical part/2(Electrical Torque)
  Convert rad/s to rmp/1 -> RPM/1
  StaticTfric/1 -> Mechanical part/1(Static Friction Torque)

== system dynamicsquat/Motors/DC Motor 5 ==
  Control Voltage : Inport
  Convert rad/s to rmp : Gain  Gain=60/(2*pi)
  Electrical part : Subsystem
  Mechanical part : Subsystem
  StaticTfric : Constant  Value=0
  Thrust : Outport  VectorParamsAs1DForOutWhenUnconnected=off
  RPM : Outport  Port=2  VectorParamsAs1DForOutWhenUnconnected=off
  ESC Current : Outport  Port=3  VectorParamsAs1DForOutWhenUnconnected=off
  Torque : Outport  Port=4  VectorParamsAs1DForOutWhenUnconnected=off
  wires:
  StaticTfric/1 -> Mechanical part/1(Static Friction Torque)
  Convert rad/s to rmp/1 -> RPM/1
  Electrical part/1(Electrical Torque) -> Mechanical part/2(Electrical Torque)
  Mechanical part/1(w angular speed) -> Electrical part/2(w angular speed), Convert rad/s to rmp/1
  Mechanical part/2(Thrust) -> Thrust/1
  Electrical part/2(current) -> ESC Current/1
  Control Voltage/1 -> Electrical part/1(ESC voltage)
  Mechanical part/3(Torque) -> Torque/1

== system dynamicsquat/Motors/DC Motor 6 ==
  Control Voltage : Inport
  Convert rad/s to rmp : Gain  Gain=60/(2*pi)
  Electrical part : Subsystem
  Mechanical part : Subsystem
  StaticTfric : Constant  Value=0
  Thrust : Outport  VectorParamsAs1DForOutWhenUnconnected=off
  RPM : Outport  Port=2  VectorParamsAs1DForOutWhenUnconnected=off
  ESC Current : Outport  Port=3  VectorParamsAs1DForOutWhenUnconnected=off
  Torque : Outport  Port=4  VectorParamsAs1DForOutWhenUnconnected=off
  wires:
  Mechanical part/3(Torque) -> Torque/1
  Control Voltage/1 -> Electrical part/1(ESC voltage)
  Electrical part/2(current) -> ESC Current/1
  Mechanical part/2(Thrust) -> Thrust/1
  Mechanical part/1(w angular speed) -> Convert rad/s to rmp/1, Electrical part/2(w angular speed)
  Electrical part/1(Electrical Torque) -> Mechanical part/2(Electrical Torque)
  Convert rad/s to rmp/1 -> RPM/1
  StaticTfric/1 -> Mechanical part/1(Static Friction Torque)

== system dynamicsquat/Motors/DC Motor 7 ==
  Control Voltage : Inport
  Convert rad/s to rmp : Gain  Gain=60/(2*pi)
  Electrical part : Subsystem
  Mechanical part : Subsystem
  StaticTfric : Constant  Value=0
  Thrust : Outport  VectorParamsAs1DForOutWhenUnconnected=off
  RPM : Outport  Port=2  VectorParamsAs1DForOutWhenUnconnected=off
  ESC Current : Outport  Port=3  VectorParamsAs1DForOutWhenUnconnected=off
  Torque : Outport  Port=4  VectorParamsAs1DForOutWhenUnconnected=off
  wires:
  StaticTfric/1 -> Mechanical part/1(Static Friction Torque)
  Convert rad/s to rmp/1 -> RPM/1
  Electrical part/1(Electrical Torque) -> Mechanical part/2(Electrical Torque)
  Mechanical part/1(w angular speed) -> Electrical part/2(w angular speed), Convert rad/s to rmp/1
  Mechanical part/2(Thrust) -> Thrust/1
  Electrical part/2(current) -> ESC Current/1
  Control Voltage/1 -> Electrical part/1(ESC voltage)
  Mechanical part/3(Torque) -> Torque/1

== system dynamicsquat/Motors/DC Motor 8 ==
  Control Voltage : Inport
  Convert rad/s to rmp : Gain  Gain=60/(2*pi)
  Electrical part : Subsystem
  Mechanical part : Subsystem
  StaticTfric : Constant  Value=0
  Thrust : Outport  VectorParamsAs1DForOutWhenUnconnected=off
  RPM : Outport  Port=2  VectorParamsAs1DForOutWhenUnconnected=off
  ESC Current : Outport  Port=3  VectorParamsAs1DForOutWhenUnconnected=off
  Torque : Outport  Port=4  VectorParamsAs1DForOutWhenUnconnected=off
  wires:
  Mechanical part/3(Torque) -> Torque/1
  Control Voltage/1 -> Electrical part/1(ESC voltage)
  Electrical part/2(current) -> ESC Current/1
  Mechanical part/2(Thrust) -> Thrust/1
  Mechanical part/1(w angular speed) -> Convert rad/s to rmp/1, Electrical part/2(w angular speed)
  Electrical part/1(Electrical Torque) -> Mechanical part/2(Electrical Torque)
  Convert rad/s to rmp/1 -> RPM/1
  StaticTfric/1 -> Mechanical part/1(Static Friction Torque)

== system dynamicsquat/Position//Velocity controllers/PD_Phi_des ==
  Ydot_ref : Inport
  Ydot : Inport  Port=2
  Add1 : Sum  Inputs=+-
  Gain : Gain  Gain=0.1
  Saturation in radians : Saturate  UpperLimit=octomodel.maxangle*pi/180  LowerLimit=-octomodel.maxangle*pi/180
  torque orientation : Gain  Gain=-1
  Phi_ref : Outport  VectorParamsAs1DForOutWhenUnconnected=off
  wires:
  Saturation in radians/1 -> Phi_ref/1
  Ydot_ref/1 -> Add1/1
  Ydot/1 -> Add1/2
  Add1/1 -> Gain/1
  Gain/1 -> torque orientation/1
  torque orientation/1 -> Saturation in radians/1

== system dynamicsquat/Position//Velocity controllers/PD_Theta_des ==
  Xdot_ref : Inport
  Xdot : Inport  Port=2
  Add1 : Sum  Inputs=+-
  Gain : Gain  Gain=0.1
  Saturation in radians1 : Saturate  UpperLimit=octomodel.maxangle*pi/180  LowerLimit=-octomodel.maxangle*pi/180
  Theta_ref : Outport  VectorParamsAs1DForOutWhenUnconnected=off
  wires:
  Xdot_ref/1 -> Add1/1
  Xdot/1 -> Add1/2
  Add1/1 -> Gain/1
  Saturation in radians1/1 -> Theta_ref/1
  Gain/1 -> Saturation in radians1/1

== system dynamicsquat/Position//Velocity controllers/Velocity controller Z ==
  z_velref : Inport
  z_vel : Inport  Port=2
  Add : Sum
  Add1 : Sum  Inputs=+-
  Constant2 : Constant  Value=octomodel.g*octomodel.mass
  Gain : Gain  Gain=25
  Thrust : Outport
  wires:
  z_velref/1 -> Add1/1
  Constant2/1 -> Add/2
  z_vel/1 -> Add1/2
  Add1/1 -> Gain/1
  Add/1 -> Thrust/1
  Gain/1 -> Add/1

== system dynamicsquat/Motors/DC Motor 1/Electrical part ==
  ESC voltage : Inport
  w angular speed : Inport  Port=2
  1/R : Gain  Gain=1/Motor.Req
  Ke (Torque constant)1 : Gain  Gain=Motor.Ke_eq
  Kt (Torque constant) Kt=Ke for an ideal square wave motor : Gain  Gain=Motor.Ke_eq
  Saturation : Saturate  UpperLimit=38  LowerLimit=0
  Sum : Sum  Inputs=|+-
  Electrical Torque : Outport  VectorParamsAs1DForOutWhenUnconnected=off
  current : Outport  Port=2  VectorParamsAs1DForOutWhenUnconnected=off
  wires:
  1/R/1 -> Saturation/1  "current i"
  Sum/1 -> 1/R/1
  Kt (Torque constant) Kt=Ke for an ideal square wave motor/1 -> Electrical Torque/1
  Ke (Torque constant)1/1 -> Sum/2
  ESC voltage/1 -> Sum/1
  w angular speed/1 -> Ke (Torque constant)1/1
  Saturation/1 -> Kt (Torque constant) Kt=Ke for an ideal square wave motor/1, current/1

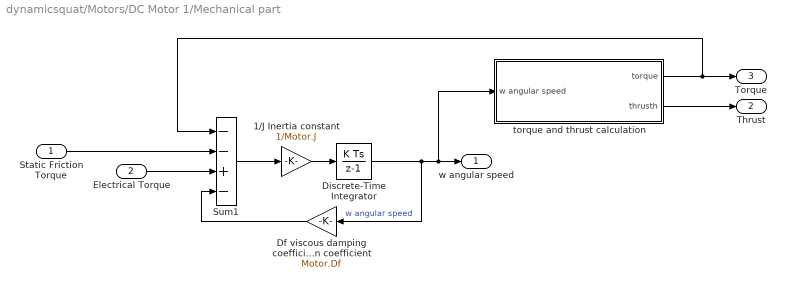
== system dynamicsquat/Motors/DC Motor 1/Mechanical part ==
  Static Friction Torque : Inport
  Electrical Torque : Inport  Port=2
  1/J Inertia constant : Gain  Gain=1/Motor.J
  "Df viscous damping coefficient Dynamic Friction coefficient " : Gain  Gain=Motor.Df
  Discrete-Time Integrator : DiscreteIntegrator  gainval=1  InitialCondition=IC.w1  SampleTime=octomodel.sampletime  ICPrevOutput=DiscIntNeverNeededParam  ICPrevScaledInput=DiscIntNeverNeededParam
  Sum1 : Sum  Inputs=--+-
  torque and thrust calculation : Subsystem
  w angular speed : Outport  VectorParamsAs1DForOutWhenUnconnected=off
  Thrust : Outport  Port=2  VectorParamsAs1DForOutWhenUnconnected=off
  Torque : Outport  Port=3  VectorParamsAs1DForOutWhenUnconnected=off
  wires:
  1/J Inertia constant/1 -> Discrete-Time Integrator/1
  Static Friction Torque/1 -> Sum1/2
  "Df viscous damping coefficient Dynamic Friction coefficient "/1 -> Sum1/4
  Discrete-Time Integrator/1 -> w angular speed/1, torque and thrust calculation/1(w angular speed), "Df viscous damping coefficient Dynamic Friction coefficient "/1  "w angular speed"
  Sum1/1 -> 1/J Inertia constant/1
  Electrical Torque/1 -> Sum1/3
  torque and thrust calculation/2(thrusth) -> Thrust/1
  torque and thrust calculation/1(torque) -> Sum1/1, Torque/1

== system dynamicsquat/Motors/DC Motor 2/Electrical part ==
  ESC voltage : Inport
  w angular speed : Inport  Port=2
  1/R : Gain  Gain=1/Motor.Req
  Ke (Torque constant)1 : Gain  Gain=Motor.Ke_eq
  Kt (Torque constant) Kt=Ke for an ideal square wave motor : Gain  Gain=Motor.Ke_eq
  Saturation : Saturate  UpperLimit=38  LowerLimit=0
  Sum : Sum  Inputs=|+-
  Electrical Torque : Outport  VectorParamsAs1DForOutWhenUnconnected=off
  current : Outport  Port=2  VectorParamsAs1DForOutWhenUnconnected=off
  wires:
  w angular speed/1 -> Ke (Torque constant)1/1
  ESC voltage/1 -> Sum/1
  Ke (Torque constant)1/1 -> Sum/2
  Kt (Torque constant) Kt=Ke for an ideal square wave motor/1 -> Electrical Torque/1
  Sum/1 -> 1/R/1
  1/R/1 -> Saturation/1  "current i"
  Saturation/1 -> current/1, Kt (Torque constant) Kt=Ke for an ideal square wave motor/1

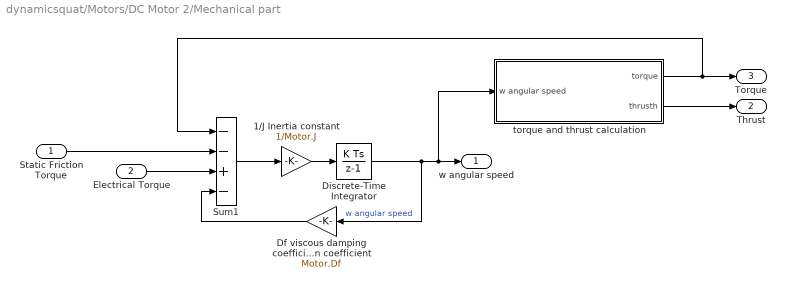
== system dynamicsquat/Motors/DC Motor 2/Mechanical part ==
  Static Friction Torque : Inport
  Electrical Torque : Inport  Port=2
  1/J Inertia constant : Gain  Gain=1/Motor.J
  "Df viscous damping coefficient Dynamic Friction coefficient " : Gain  Gain=Motor.Df
  Discrete-Time Integrator : DiscreteIntegrator  gainval=1  InitialCondition=IC.w2  SampleTime=octomodel.sampletime  ICPrevOutput=DiscIntNeverNeededParam  ICPrevScaledInput=DiscIntNeverNeededParam
  Sum1 : Sum  Inputs=--+-
  torque and thrust calculation : Subsystem
  w angular speed : Outport  VectorParamsAs1DForOutWhenUnconnected=off
  Thrust : Outport  Port=2  VectorParamsAs1DForOutWhenUnconnected=off
  Torque : Outport  Port=3  VectorParamsAs1DForOutWhenUnconnected=off
  wires:
  torque and thrust calculation/1(torque) -> Torque/1, Sum1/1
  torque and thrust calculation/2(thrusth) -> Thrust/1
  Electrical Torque/1 -> Sum1/3
  Sum1/1 -> 1/J Inertia constant/1
  Discrete-Time Integrator/1 -> "Df viscous damping coefficient Dynamic Friction coefficient "/1, torque and thrust calculation/1(w angular speed), w angular speed/1  "w angular speed"
  "Df viscous damping coefficient Dynamic Friction coefficient "/1 -> Sum1/4
  Static Friction Torque/1 -> Sum1/2
  1/J Inertia constant/1 -> Discrete-Time Integrator/1

== system dynamicsquat/Motors/DC Motor 3/Electrical part ==
  ESC voltage : Inport
  w angular speed : Inport  Port=2
  1/R : Gain  Gain=1/Motor.Req
  Ke (Torque constant)1 : Gain  Gain=Motor.Ke_eq
  Kt (Torque constant) Kt=Ke for an ideal square wave motor : Gain  Gain=Motor.Ke_eq
  Saturation : Saturate  UpperLimit=38  LowerLimit=0
  Sum : Sum  Inputs=|+-
  Electrical Torque : Outport  VectorParamsAs1DForOutWhenUnconnected=off
  current : Outport  Port=2  VectorParamsAs1DForOutWhenUnconnected=off
  wires:
  1/R/1 -> Saturation/1  "current i"
  Sum/1 -> 1/R/1
  Kt (Torque constant) Kt=Ke for an ideal square wave motor/1 -> Electrical Torque/1
  Ke (Torque constant)1/1 -> Sum/2
  ESC voltage/1 -> Sum/1
  w angular speed/1 -> Ke (Torque constant)1/1
  Saturation/1 -> Kt (Torque constant) Kt=Ke for an ideal square wave motor/1, current/1

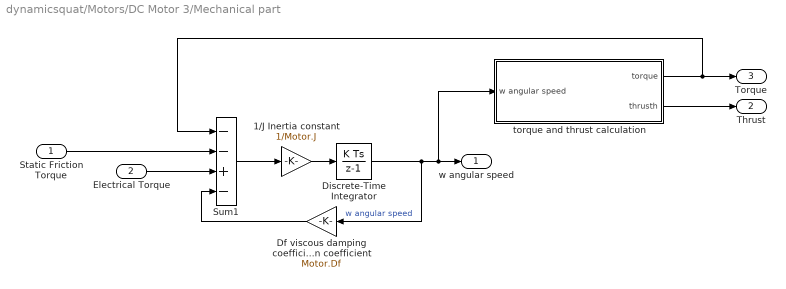
== system dynamicsquat/Motors/DC Motor 3/Mechanical part ==
  Static Friction Torque : Inport
  Electrical Torque : Inport  Port=2
  1/J Inertia constant : Gain  Gain=1/Motor.J
  "Df viscous damping coefficient Dynamic Friction coefficient " : Gain  Gain=Motor.Df
  Discrete-Time Integrator : DiscreteIntegrator  gainval=1  InitialCondition=IC.w3  SampleTime=octomodel.sampletime  ICPrevOutput=DiscIntNeverNeededParam  ICPrevScaledInput=DiscIntNeverNeededParam
  Sum1 : Sum  Inputs=--+-
  torque and thrust calculation : Subsystem
  w angular speed : Outport  VectorParamsAs1DForOutWhenUnconnected=off
  Thrust : Outport  Port=2  VectorParamsAs1DForOutWhenUnconnected=off
  Torque : Outport  Port=3  VectorParamsAs1DForOutWhenUnconnected=off
  wires:
  1/J Inertia constant/1 -> Discrete-Time Integrator/1
  Static Friction Torque/1 -> Sum1/2
  "Df viscous damping coefficient Dynamic Friction coefficient "/1 -> Sum1/4
  Discrete-Time Integrator/1 -> w angular speed/1, torque and thrust calculation/1(w angular speed), "Df viscous damping coefficient Dynamic Friction coefficient "/1  "w angular speed"
  Sum1/1 -> 1/J Inertia constant/1
  Electrical Torque/1 -> Sum1/3
  torque and thrust calculation/2(thrusth) -> Thrust/1
  torque and thrust calculation/1(torque) -> Sum1/1, Torque/1

== system dynamicsquat/Motors/DC Motor 4/Electrical part ==
  ESC voltage : Inport
  w angular speed : Inport  Port=2
  1/R : Gain  Gain=1/Motor.Req
  Ke (Torque constant)1 : Gain  Gain=Motor.Ke_eq
  Kt (Torque constant) Kt=Ke for an ideal square wave motor : Gain  Gain=Motor.Ke_eq
  Saturation : Saturate  UpperLimit=38  LowerLimit=0
  Sum : Sum  Inputs=|+-
  Electrical Torque : Outport  VectorParamsAs1DForOutWhenUnconnected=off
  current : Outport  Port=2  VectorParamsAs1DForOutWhenUnconnected=off
  wires:
  w angular speed/1 -> Ke (Torque constant)1/1
  ESC voltage/1 -> Sum/1
  Ke (Torque constant)1/1 -> Sum/2
  Kt (Torque constant) Kt=Ke for an ideal square wave motor/1 -> Electrical Torque/1
  Sum/1 -> 1/R/1
  1/R/1 -> Saturation/1  "current i"
  Saturation/1 -> current/1, Kt (Torque constant) Kt=Ke for an ideal square wave motor/1

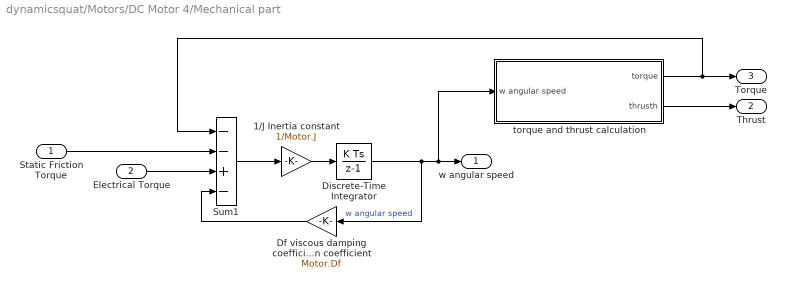
== system dynamicsquat/Motors/DC Motor 4/Mechanical part ==
  Static Friction Torque : Inport
  Electrical Torque : Inport  Port=2
  1/J Inertia constant : Gain  Gain=1/Motor.J
  "Df viscous damping coefficient Dynamic Friction coefficient " : Gain  Gain=Motor.Df
  Discrete-Time Integrator : DiscreteIntegrator  gainval=1  InitialCondition=IC.w4  SampleTime=octomodel.sampletime  ICPrevOutput=DiscIntNeverNeededParam  ICPrevScaledInput=DiscIntNeverNeededParam
  Sum1 : Sum  Inputs=--+-
  torque and thrust calculation : Subsystem
  w angular speed : Outport  VectorParamsAs1DForOutWhenUnconnected=off
  Thrust : Outport  Port=2  VectorParamsAs1DForOutWhenUnconnected=off
  Torque : Outport  Port=3  VectorParamsAs1DForOutWhenUnconnected=off
  wires:
  torque and thrust calculation/1(torque) -> Torque/1, Sum1/1
  torque and thrust calculation/2(thrusth) -> Thrust/1
  Electrical Torque/1 -> Sum1/3
  Sum1/1 -> 1/J Inertia constant/1
  Discrete-Time Integrator/1 -> "Df viscous damping coefficient Dynamic Friction coefficient "/1, torque and thrust calculation/1(w angular speed), w angular speed/1  "w angular speed"
  "Df viscous damping coefficient Dynamic Friction coefficient "/1 -> Sum1/4
  Static Friction Torque/1 -> Sum1/2
  1/J Inertia constant/1 -> Discrete-Time Integrator/1

== system dynamicsquat/Motors/DC Motor 5/Electrical part ==
  ESC voltage : Inport
  w angular speed : Inport  Port=2
  1/R : Gain  Gain=1/Motor.Req
  Ke (Torque constant)1 : Gain  Gain=Motor.Ke_eq
  Kt (Torque constant) Kt=Ke for an ideal square wave motor : Gain  Gain=Motor.Ke_eq
  Saturation : Saturate  UpperLimit=38  LowerLimit=0
  Sum : Sum  Inputs=|+-
  Electrical Torque : Outport  VectorParamsAs1DForOutWhenUnconnected=off
  current : Outport  Port=2  VectorParamsAs1DForOutWhenUnconnected=off
  wires:
  1/R/1 -> Saturation/1  "current i"
  Sum/1 -> 1/R/1
  Kt (Torque constant) Kt=Ke for an ideal square wave motor/1 -> Electrical Torque/1
  Ke (Torque constant)1/1 -> Sum/2
  ESC voltage/1 -> Sum/1
  w angular speed/1 -> Ke (Torque constant)1/1
  Saturation/1 -> Kt (Torque constant) Kt=Ke for an ideal square wave motor/1, current/1

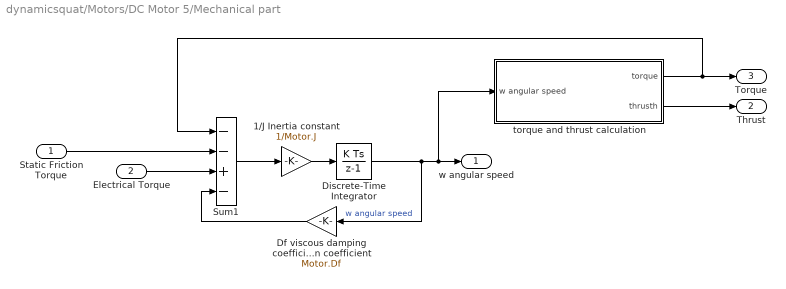
== system dynamicsquat/Motors/DC Motor 5/Mechanical part ==
  Static Friction Torque : Inport
  Electrical Torque : Inport  Port=2
  1/J Inertia constant : Gain  Gain=1/Motor.J
  "Df viscous damping coefficient Dynamic Friction coefficient " : Gain  Gain=Motor.Df
  Discrete-Time Integrator : DiscreteIntegrator  gainval=1  InitialCondition=IC.w5  SampleTime=octomodel.sampletime  ICPrevOutput=DiscIntNeverNeededParam  ICPrevScaledInput=DiscIntNeverNeededParam
  Sum1 : Sum  Inputs=--+-
  torque and thrust calculation : Subsystem
  w angular speed : Outport  VectorParamsAs1DForOutWhenUnconnected=off
  Thrust : Outport  Port=2  VectorParamsAs1DForOutWhenUnconnected=off
  Torque : Outport  Port=3  VectorParamsAs1DForOutWhenUnconnected=off
  wires:
  1/J Inertia constant/1 -> Discrete-Time Integrator/1
  Static Friction Torque/1 -> Sum1/2
  "Df viscous damping coefficient Dynamic Friction coefficient "/1 -> Sum1/4
  Discrete-Time Integrator/1 -> w angular speed/1, torque and thrust calculation/1(w angular speed), "Df viscous damping coefficient Dynamic Friction coefficient "/1  "w angular speed"
  Sum1/1 -> 1/J Inertia constant/1
  Electrical Torque/1 -> Sum1/3
  torque and thrust calculation/2(thrusth) -> Thrust/1
  torque and thrust calculation/1(torque) -> Sum1/1, Torque/1

== system dynamicsquat/Motors/DC Motor 6/Electrical part ==
  ESC voltage : Inport
  w angular speed : Inport  Port=2
  1/R : Gain  Gain=1/Motor.Req
  Ke (Torque constant)1 : Gain  Gain=Motor.Ke_eq
  Kt (Torque constant) Kt=Ke for an ideal square wave motor : Gain  Gain=Motor.Ke_eq
  Saturation : Saturate  UpperLimit=38  LowerLimit=0
  Sum : Sum  Inputs=|+-
  Electrical Torque : Outport  VectorParamsAs1DForOutWhenUnconnected=off
  current : Outport  Port=2  VectorParamsAs1DForOutWhenUnconnected=off
  wires:
  w angular speed/1 -> Ke (Torque constant)1/1
  ESC voltage/1 -> Sum/1
  Ke (Torque constant)1/1 -> Sum/2
  Kt (Torque constant) Kt=Ke for an ideal square wave motor/1 -> Electrical Torque/1
  Sum/1 -> 1/R/1
  1/R/1 -> Saturation/1  "current i"
  Saturation/1 -> current/1, Kt (Torque constant) Kt=Ke for an ideal square wave motor/1

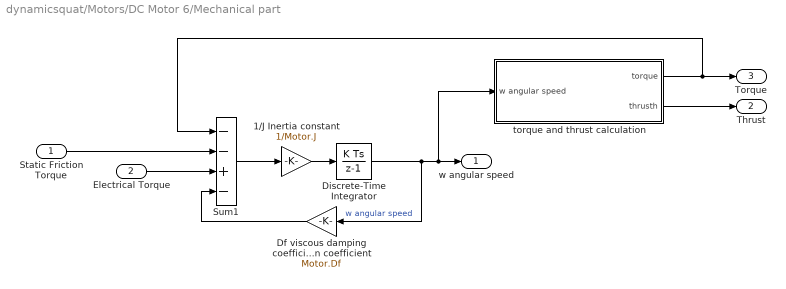
== system dynamicsquat/Motors/DC Motor 6/Mechanical part ==
  Static Friction Torque : Inport
  Electrical Torque : Inport  Port=2
  1/J Inertia constant : Gain  Gain=1/Motor.J
  "Df viscous damping coefficient Dynamic Friction coefficient " : Gain  Gain=Motor.Df
  Discrete-Time Integrator : DiscreteIntegrator  gainval=1  InitialCondition=IC.w6  SampleTime=octomodel.sampletime  ICPrevOutput=DiscIntNeverNeededParam  ICPrevScaledInput=DiscIntNeverNeededParam
  Sum1 : Sum  Inputs=--+-
  torque and thrust calculation : Subsystem
  w angular speed : Outport  VectorParamsAs1DForOutWhenUnconnected=off
  Thrust : Outport  Port=2  VectorParamsAs1DForOutWhenUnconnected=off
  Torque : Outport  Port=3  VectorParamsAs1DForOutWhenUnconnected=off
  wires:
  torque and thrust calculation/1(torque) -> Torque/1, Sum1/1
  torque and thrust calculation/2(thrusth) -> Thrust/1
  Electrical Torque/1 -> Sum1/3
  Sum1/1 -> 1/J Inertia constant/1
  Discrete-Time Integrator/1 -> "Df viscous damping coefficient Dynamic Friction coefficient "/1, torque and thrust calculation/1(w angular speed), w angular speed/1  "w angular speed"
  "Df viscous damping coefficient Dynamic Friction coefficient "/1 -> Sum1/4
  Static Friction Torque/1 -> Sum1/2
  1/J Inertia constant/1 -> Discrete-Time Integrator/1

== system dynamicsquat/Motors/DC Motor 7/Electrical part ==
  ESC voltage : Inport
  w angular speed : Inport  Port=2
  1/R : Gain  Gain=1/Motor.Req
  Ke (Torque constant)1 : Gain  Gain=Motor.Ke_eq
  Kt (Torque constant) Kt=Ke for an ideal square wave motor : Gain  Gain=Motor.Ke_eq
  Saturation : Saturate  UpperLimit=38  LowerLimit=0
  Sum : Sum  Inputs=|+-
  Electrical Torque : Outport  VectorParamsAs1DForOutWhenUnconnected=off
  current : Outport  Port=2  VectorParamsAs1DForOutWhenUnconnected=off
  wires:
  1/R/1 -> Saturation/1  "current i"
  Sum/1 -> 1/R/1
  Kt (Torque constant) Kt=Ke for an ideal square wave motor/1 -> Electrical Torque/1
  Ke (Torque constant)1/1 -> Sum/2
  ESC voltage/1 -> Sum/1
  w angular speed/1 -> Ke (Torque constant)1/1
  Saturation/1 -> Kt (Torque constant) Kt=Ke for an ideal square wave motor/1, current/1

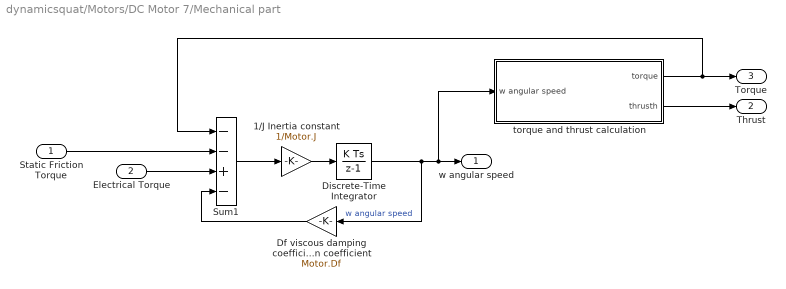
== system dynamicsquat/Motors/DC Motor 7/Mechanical part ==
  Static Friction Torque : Inport
  Electrical Torque : Inport  Port=2
  1/J Inertia constant : Gain  Gain=1/Motor.J
  "Df viscous damping coefficient Dynamic Friction coefficient " : Gain  Gain=Motor.Df
  Discrete-Time Integrator : DiscreteIntegrator  gainval=1  InitialCondition=IC.w7  SampleTime=octomodel.sampletime  ICPrevOutput=DiscIntNeverNeededParam  ICPrevScaledInput=DiscIntNeverNeededParam
  Sum1 : Sum  Inputs=--+-
  torque and thrust calculation : Subsystem
  w angular speed : Outport  VectorParamsAs1DForOutWhenUnconnected=off
  Thrust : Outport  Port=2  VectorParamsAs1DForOutWhenUnconnected=off
  Torque : Outport  Port=3  VectorParamsAs1DForOutWhenUnconnected=off
  wires:
  1/J Inertia constant/1 -> Discrete-Time Integrator/1
  Static Friction Torque/1 -> Sum1/2
  "Df viscous damping coefficient Dynamic Friction coefficient "/1 -> Sum1/4
  Discrete-Time Integrator/1 -> w angular speed/1, torque and thrust calculation/1(w angular speed), "Df viscous damping coefficient Dynamic Friction coefficient "/1  "w angular speed"
  Sum1/1 -> 1/J Inertia constant/1
  Electrical Torque/1 -> Sum1/3
  torque and thrust calculation/2(thrusth) -> Thrust/1
  torque and thrust calculation/1(torque) -> Sum1/1, Torque/1

== system dynamicsquat/Motors/DC Motor 8/Electrical part ==
  ESC voltage : Inport
  w angular speed : Inport  Port=2
  1/R : Gain  Gain=1/Motor.Req
  Ke (Torque constant)1 : Gain  Gain=Motor.Ke_eq
  Kt (Torque constant) Kt=Ke for an ideal square wave motor : Gain  Gain=Motor.Ke_eq
  Saturation : Saturate  UpperLimit=38  LowerLimit=0
  Sum : Sum  Inputs=|+-
  Electrical Torque : Outport  VectorParamsAs1DForOutWhenUnconnected=off
  current : Outport  Port=2  VectorParamsAs1DForOutWhenUnconnected=off
  wires:
  w angular speed/1 -> Ke (Torque constant)1/1
  ESC voltage/1 -> Sum/1
  Ke (Torque constant)1/1 -> Sum/2
  Kt (Torque constant) Kt=Ke for an ideal square wave motor/1 -> Electrical Torque/1
  Sum/1 -> 1/R/1
  1/R/1 -> Saturation/1  "current i"
  Saturation/1 -> current/1, Kt (Torque constant) Kt=Ke for an ideal square wave motor/1

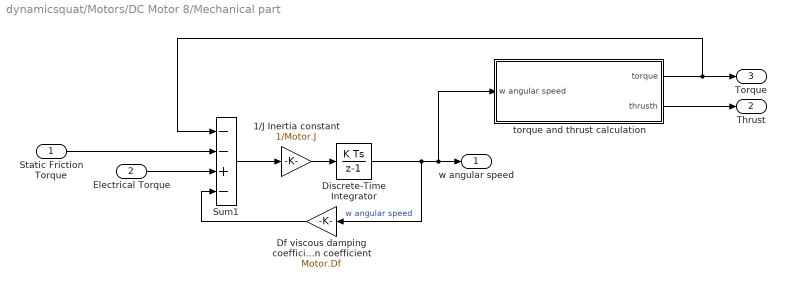
== system dynamicsquat/Motors/DC Motor 8/Mechanical part ==
  Static Friction Torque : Inport
  Electrical Torque : Inport  Port=2
  1/J Inertia constant : Gain  Gain=1/Motor.J
  "Df viscous damping coefficient Dynamic Friction coefficient " : Gain  Gain=Motor.Df
  Discrete-Time Integrator : DiscreteIntegrator  gainval=1  InitialCondition=IC.w8  SampleTime=octomodel.sampletime  ICPrevOutput=DiscIntNeverNeededParam  ICPrevScaledInput=DiscIntNeverNeededParam
  Sum1 : Sum  Inputs=--+-
  torque and thrust calculation : Subsystem
  w angular speed : Outport  VectorParamsAs1DForOutWhenUnconnected=off
  Thrust : Outport  Port=2  VectorParamsAs1DForOutWhenUnconnected=off
  Torque : Outport  Port=3  VectorParamsAs1DForOutWhenUnconnected=off
  wires:
  torque and thrust calculation/1(torque) -> Torque/1, Sum1/1
  torque and thrust calculation/2(thrusth) -> Thrust/1
  Electrical Torque/1 -> Sum1/3
  Sum1/1 -> 1/J Inertia constant/1
  Discrete-Time Integrator/1 -> "Df viscous damping coefficient Dynamic Friction coefficient "/1, torque and thrust calculation/1(w angular speed), w angular speed/1  "w angular speed"
  "Df viscous damping coefficient Dynamic Friction coefficient "/1 -> Sum1/4
  Static Friction Torque/1 -> Sum1/2
  1/J Inertia constant/1 -> Discrete-Time Integrator/1

== system dynamicsquat/Motors/DC Motor 1/Mechanical part/torque and thrust calculation ==
  w angular speed : Inport
  Convert rad/s to rmp : Gain  Gain=60/(2*pi)
  "Propeller model " : MATLAB Function  TreatAsAtomicUnit=on
  torque : Outport  VectorParamsAs1DForOutWhenUnconnected=off
  thrusth : Outport  Port=2  VectorParamsAs1DForOutWhenUnconnected=off
  wires:
  Convert rad/s to rmp/1 -> "Propeller model "/1(rpm)
  w angular speed/1 -> Convert rad/s to rmp/1
  "Propeller model "/2(thrust) -> thrusth/1
  "Propeller model "/1(torque) -> torque/1

== system dynamicsquat/Motors/DC Motor 2/Mechanical part/torque and thrust calculation ==
  w angular speed : Inport
  Convert rad/s to rmp : Gain  Gain=60/(2*pi)
  "Propeller model " : MATLAB Function  TreatAsAtomicUnit=on
  torque : Outport  VectorParamsAs1DForOutWhenUnconnected=off
  thrusth : Outport  Port=2  VectorParamsAs1DForOutWhenUnconnected=off
  wires:
  "Propeller model "/1(torque) -> torque/1
  "Propeller model "/2(thrust) -> thrusth/1
  w angular speed/1 -> Convert rad/s to rmp/1
  Convert rad/s to rmp/1 -> "Propeller model "/1(rpm)
